simulink model "PVBOOSTCPL_MPPT"  (R2015a)
settings: Solver=ode3  StartTime=0.0  StopTime=inf  FixedStep=5e-5  RelTol=1e-3
libraries: powerlib x24, simulink x3, powerlib_meascontrol x2, fuzblock x1, simulink_extras x1, re_lib x1
settings Model: CovModelRefEnable=off  Creator=Nady  LastModifiedBy=ga63vey
settings DataIOCC: SaveFormat=Dataset
settings HardwareCC: ProdBitPerPointer=64  ProdLargestAtomicFloat=Float  ProdIntDivRoundTo=Zero  ProdEndianess=LittleEndian  ProdHWDeviceType=Specified
settings GRTTargetCC: GeneratePreprocessorConditionals=Use local settings

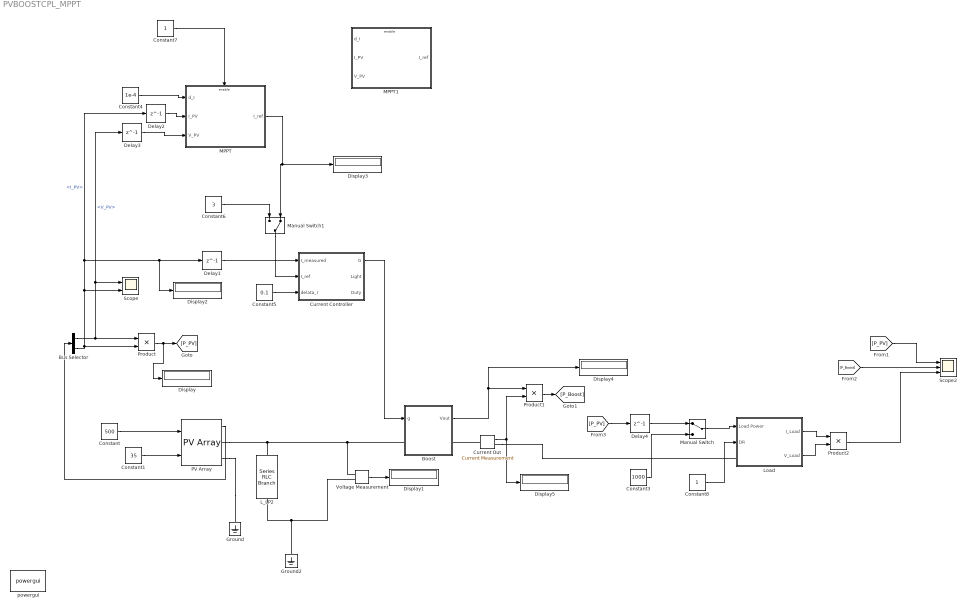
== system PVBOOSTCPL_MPPT ==
  Boost : Subsystem
  Bus Selector : BusSelector  OutputSignals=V_PV,I_PV
  Constant : Constant  Value=500
  Constant1 : Constant  Value=35
  Constant3 : Constant  Value=1000
  Constant4 : Constant  Value=1e-4
  Constant5 : Constant  Value=0.1
  Constant6 : Constant  Value=3
  Constant7 : Constant
  Constant8 : Constant
  Current Controller : Subsystem  TreatAsAtomicUnit=on
  Current Out : powerlib/Measurements/Current Measurement  PhasorSimulation=off  OutputType=Complex  PSBequivalent=0
  Delay{1..4} (4 alike) : Delay  DelayLength=1  InitialCondition=0
  Display{,1..5} (6 alike) : Display
  Ground : powerlib/Elements/Ground  LConnTagsString=a
  Ground2 : powerlib/Elements/Ground  LConnTagsString=a
  L_LP2 : powerlib/Elements/Series RLC Branch  LConnTagsString=__new0  RConnTagsString=__new0  BranchType=RC  Resistance=0.5  Inductance=0.0164  SetiL0=off  InitialCurrent=0  Capacitance=0.1  Setx0=off  InitialVoltage=0  Measurements=None
  Load : Subsystem
  MPPT : Subsystem
  MPPT1 : Subsystem
  Manual Switch : ManualSwitch
  Manual Switch1 : ManualSwitch  CurrentSetting=0
  PV Array : re_lib/Solar/PV Array  Npar=1  Nser=1  PlotType=array @ 1000 W/m2 & specified temperatures  S_vec="[ 1000  500  100 ]"  Temp_C_vec=[35]  ModuleName=Sun Earth Solar Power TDB125x125-36-P 80W  PlotWhenSelected=off  Pm=80.004  Ncell=36  Voc=21.9  Isc=5  Vm=17.7  Im=4.52  beta_Voc_pc=-0.32  alpha_Isc_pc=0.04  beta_Voc=-0.07008  alpha_Isc=0.002  IL=5.0238  I0=3.6974e-11  nI=0.92596  Rsh=70.2892  Rs=0.35567  BAL=off  Tc=1e-6  Tfilter=5e-5
  Product : Product
  Product1 : Product
  Product2 : Product
  Scope : Scope  NumInputPorts=2
      settings: YMin=-4.3176~-0.64549  YMax=38.86394~7.07339
  Scope2 : Scope  NumInputPorts=3
      settings: YMin=57~58~57  YMax=64~64~64  SaveName=ScopeData2
  Voltage Measurement : powerlib/Measurements/Voltage Measurement  PhasorSimulation=off  OutputType=Complex  PSBequivalent=0
  powergui : powerlib/powergui  Priority=1  SimulationMode=Discrete  SolverType=Tustin  SampleTime=50e-6  frequency=60  SPID=off  DisableSnubberDevices=off  DisableRonSwitches=off  DisableVfSwitches=off  SwTol=0  DisplayEquations=off  Interpol=off  methode=off  Ts=10  FunctionMessages=off  echomessages=off  HookPort=off  EnableUseOfTLC=off  x0status=blocks  frequencyindice=0  Pbase=100e6  ErrMax=1e-4  Iterations=50  UnitsV=kV  UnitsW=MW  buscounter=0  RestoreLinks=warning  ResistiveCurrentMeasurement=off  Frange=[0:2:500]  Ylog=off  Xlog=on  ShowGrid=off  save=off  variable=ZData  structure=0  ZoomFFT=off  StartTime=0.0  cycles=1  DisplayStyle=1  fundamental=60  FreqAxis=off  MaxFrequency=1000  frequencyindicesteady=1  RmsSteady=1  display=off
  wires:
  Constant/1 -> PV Array/1
  Constant1/1 -> PV Array/2
  PV Array/1 -> Bus Selector/1
  Bus Selector/1 -> Delay3/1, Scope/1, Product/1  "<V_PV>"
  Bus Selector/2 -> Delay2/1, Display2/1, Delay1/1, Scope/2, Product/2  "<I_PV>"
  Boost/1(Vout) -> Display4/1, Product1/1
  Current Out/1 -> Product1/2, Display5/1
  Product/1 -> Display/1, [P_PV]
  Product1/1 -> [P_Boost]
  Manual Switch/1 -> Load/1(Load Power)
  Constant3/1 -> Manual Switch/2
  [P_PV] -> Delay4/1
  Voltage Measurement/1 -> Display1/1
  Constant5/1 -> Current Controller/3(delata_I)
  Delay1/1 -> Current Controller/1(I_measured)
  Constant4/1 -> MPPT/1(d_I)
  Delay2/1 -> MPPT/2(I_PV)
  Delay3/1 -> MPPT/3(V_PV)
  Delay4/1 -> Manual Switch/1
  MPPT/1(I_ref) -> Display3/1, Manual Switch1/2
  Constant7/1 -> MPPT/Enable
  Constant6/1 -> Manual Switch1/1
  Manual Switch1/1 -> Current Controller/2(I_ref)
  Constant8/1 -> Load/2(DR)
  [P_PV] -> Scope2/1
  [P_Boost] -> Scope2/2
  Load/1(I_Load) -> Product2/1
  Load/2(V_Load) -> Product2/2
  Product2/1 -> Scope2/3
  Current Controller/1(G) -> Boost/1(g)
  connections:
  PV Array/RConn2 -- Ground/LConn1
  Current Out/LConn1 -- Boost/RConn1
  Ground2/LConn1 -- Voltage Measurement/LConn2 -- L_LP2/LConn1
  Current Out/RConn1 -- Load/LConn1
  PV Array/RConn1 -- Voltage Measurement/LConn1 -- Boost/LConn1 -- L_LP2/RConn1

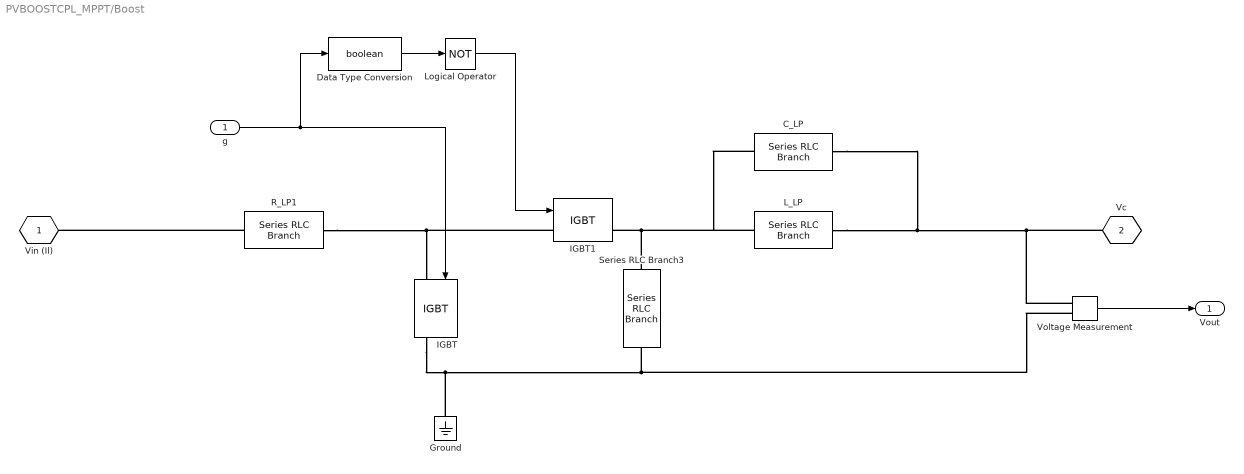
== system PVBOOSTCPL_MPPT/Boost ==
  g : Inport
  C_LP : powerlib/Elements/Series RLC Branch  LConnTagsString=__new0  RConnTagsString=__new0  BranchType=R  Resistance=10  Inductance=1e-3  SetiL0=off  InitialCurrent=0  Capacitance=0.004  Setx0=off  InitialVoltage=0  Measurements=None
  Data Type Conversion : DataTypeConversion  OutDataTypeStr=boolean
  Ground : powerlib/Elements/Ground  LConnTagsString=a
  IGBT : powerlib/Power Electronics/IGBT  Ron=0.001  Lon=0  Vf=1  Tf=1e-6  Tt=2e-6  IC=0  Rs=1e5  Cs=inf  Measurements=on
  IGBT1 : powerlib/Power Electronics/IGBT  Ron=0.001  Lon=0  Vf=1  Tf=1e-6  Tt=2e-6  IC=0  Rs=1e5  Cs=inf  Measurements=on
  L_LP : powerlib/Elements/Series RLC Branch  LConnTagsString=__new0  RConnTagsString=__new0  BranchType=L  Resistance=0.01  Inductance=0.0164  SetiL0=off  InitialCurrent=0  Capacitance=6e-2  Setx0=off  InitialVoltage=0  Measurements=None
  Logical Operator : Logic  Operator=NOT  AllPortsSameDT=off  OutDataTypeStr=boolean
  R_LP1 : powerlib/Elements/Series RLC Branch  LConnTagsString=__new0  RConnTagsString=__new0  BranchType=L  Resistance=0.01  Inductance=7e-3  SetiL0=off  InitialCurrent=0  Capacitance=6e-2  Setx0=off  InitialVoltage=0  Measurements=None
  Series RLC Branch3 : powerlib/Elements/Series RLC Branch  LConnTagsString=__new0  RConnTagsString=__new0  BranchType=RC  Resistance=0.1  Inductance=1e-3  SetiL0=off  InitialCurrent=0  Capacitance=6e-3  Setx0=off  InitialVoltage=0  Measurements=None
  Voltage Measurement : powerlib/Measurements/Voltage Measurement  PhasorSimulation=off  OutputType=Complex  PSBequivalent=0
  Vin (Il) : PMIOPort  Tag=PMCPort  Port=1  Side=Left
  Vc : PMIOPort  Tag=PMCPort  Port=2  Side=Right
  Vout : Outport
  wires:
  Voltage Measurement/1 -> Vout/1
  Data Type Conversion/1 -> Logical Operator/1
  Logical Operator/1 -> IGBT1/1
  g/1 -> Data Type Conversion/1, IGBT/1
  connections:
  IGBT/RConn1 -- Ground/LConn1 -- Voltage Measurement/LConn2 -- Series RLC Branch3/RConn1
  IGBT1/LConn1 -- R_LP1/LConn1 -- IGBT/LConn1
  R_LP1/RConn1 -- Vin (Il)/RConn1
  L_LP/LConn1 -- C_LP/LConn1 -- Voltage Measurement/LConn1 -- Vc/RConn1
  Series RLC Branch3/LConn1 -- C_LP/RConn1 -- L_LP/RConn1 -- IGBT1/RConn1

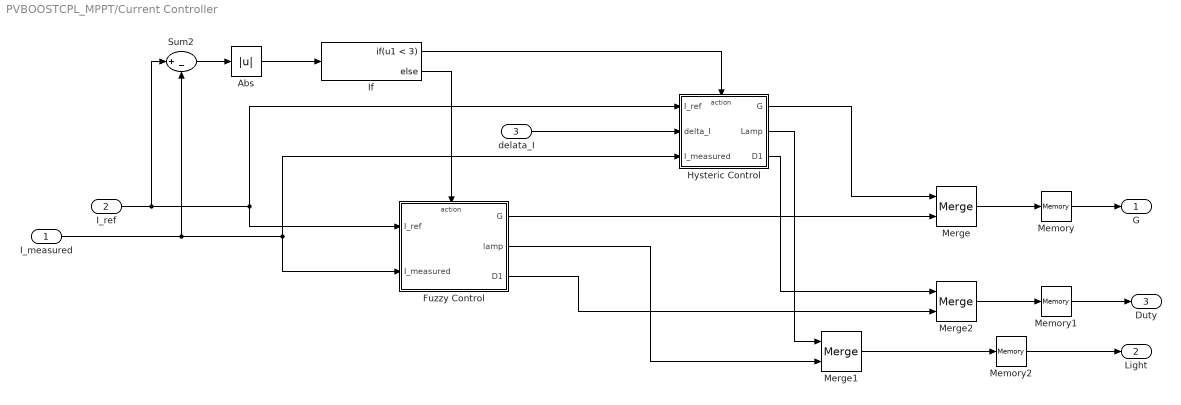
== system PVBOOSTCPL_MPPT/Current Controller ==
  I_measured : Inport  SampleTime=5e-5
  I_ref : Inport  Port=2  SampleTime=5e-5
  delata_I : Inport  Port=3
  Abs : Abs
  Fuzzy Control : Subsystem  TreatAsAtomicUnit=on
  Hysteric Control : Subsystem  TreatAsAtomicUnit=on
  If : If  IfExpression=u1 < 3
  Memory : Memory
  Memory1 : Memory
  Memory2 : Memory
  Merge : Merge
  Merge1 : Merge
  Merge2 : Merge
  Sum2 : Sum  Inputs=|+-
  G : Outport
  Light : Outport  Port=2
  Duty : Outport  Port=3
  wires:
  If/1 -> Hysteric Control/Action
  If/2 -> Fuzzy Control/Action
  I_ref/1 -> Sum2/1, Hysteric Control/1(I_ref), Fuzzy Control/1(I_ref)
  I_measured/1 -> Hysteric Control/3(I_measured), Fuzzy Control/2(I_measured), Sum2/2
  Fuzzy Control/1(G) -> Merge/2
  Merge/1 -> Memory/1
  delata_I/1 -> Hysteric Control/2(delta_I)
  Hysteric Control/1(G) -> Merge/1
  Hysteric Control/2(Lamp) -> Merge1/1
  Fuzzy Control/2(lamp) -> Merge1/2
  Merge1/1 -> Memory2/1
  Sum2/1 -> Abs/1
  Abs/1 -> If/1
  Fuzzy Control/3(D1) -> Merge2/2
  Merge2/1 -> Memory1/1
  Hysteric Control/3(D1) -> Merge2/1
  Memory/1 -> G/1
  Memory1/1 -> Duty/1
  Memory2/1 -> Light/1

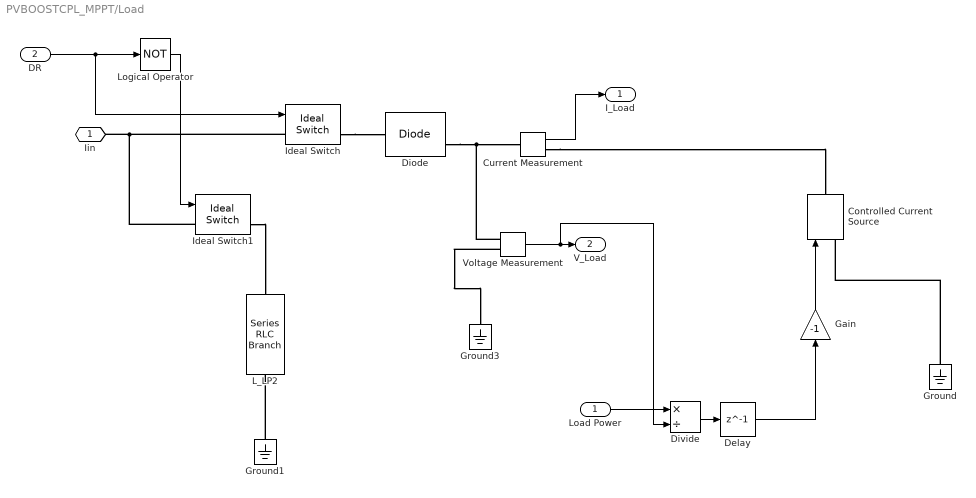
== system PVBOOSTCPL_MPPT/Load ==
  Load Power : Inport
  DR : Inport  Port=2
  Controlled Current Source : powerlib/Electrical Sources/Controlled Current Source  Initialize=on  Source_Type=AC  Amplitude=0  Phase=0  Frequency=0  Measurements=None
  Current Measurement : powerlib/Measurements/Current Measurement  PhasorSimulation=off  OutputType=Complex  PSBequivalent=0
  Delay : Delay  DelayLength=1
  Diode : powerlib/Power Electronics/Diode  Ron=0.001  Lon=0  Vf=0.8  IC=0  UseSnubber=off  Rs=500  Cs=250e-9  Measurements=on
  Divide : Product  Inputs=*/
  Gain : Gain  Gain=-1
  Ground : powerlib/Elements/Ground  LConnTagsString=a
  Ground1 : powerlib/Elements/Ground  LConnTagsString=a
  Ground3 : powerlib/Elements/Ground  LConnTagsString=a
  Ideal Switch : powerlib/Power Electronics/Ideal Switch  Ron=0.001  Lon=0  IC=0  Rs=1e5  Cs=inf  Measurements=on
  Ideal Switch1 : powerlib/Power Electronics/Ideal Switch  Ron=0.001  Lon=0  IC=0  Rs=1e5  Cs=inf  Measurements=on
  L_LP2 : powerlib/Elements/Series RLC Branch  LConnTagsString=__new0  RConnTagsString=__new0  BranchType=R  Resistance=1  Inductance=0.0164  SetiL0=off  InitialCurrent=0  Capacitance=0.1  Setx0=off  InitialVoltage=0  Measurements=None
  Logical Operator : Logic  Operator=NOT  AllPortsSameDT=off  OutDataTypeStr=boolean
  Voltage Measurement : powerlib/Measurements/Voltage Measurement  PhasorSimulation=off  OutputType=Complex  PSBequivalent=0
  Iin : PMIOPort  Port=1  Side=Left
  I_Load : Outport
  V_Load : Outport  Port=2
  wires:
  Current Measurement/1 -> I_Load/1
  Voltage Measurement/1 -> Divide/2, V_Load/1
  Load Power/1 -> Divide/1
  Gain/1 -> Controlled Current Source/1
  Divide/1 -> Delay/1
  Delay/1 -> Gain/1
  Logical Operator/1 -> Ideal Switch1/1
  DR/1 -> Ideal Switch/1, Logical Operator/1
  connections:
  Voltage Measurement/LConn1 -- Diode/RConn1 -- Current Measurement/LConn1
  Voltage Measurement/LConn2 -- Ground3/LConn1
  Ground/LConn1 -- Controlled Current Source/LConn1
  Current Measurement/RConn1 -- Controlled Current Source/RConn1
  Ideal Switch/LConn1 -- Ideal Switch1/LConn1 -- Iin/RConn1
  Ground1/LConn1 -- L_LP2/LConn1
  Ideal Switch/RConn1 -- Diode/LConn1
  Ideal Switch1/RConn1 -- L_LP2/RConn1

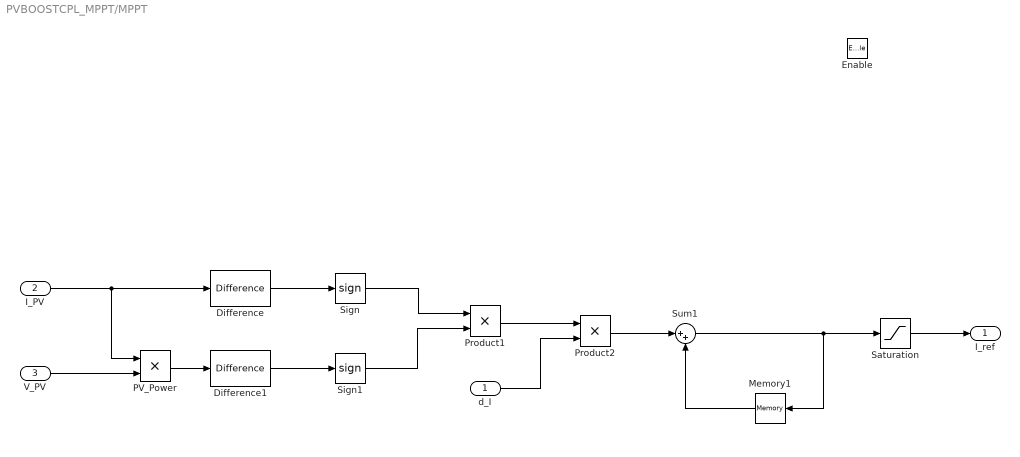
== system PVBOOSTCPL_MPPT/MPPT ==
  d_I : Inport
  I_PV : Inport  Port=2
  V_PV : Inport  Port=3
  Enable : EnablePort
  Difference : simulink/Discrete/Difference  ICPrevInput=0.0  InputProcessing=Inherited  OutMin=[]  OutMax=[]  OutDataType=fixdt(1, 16)  OutScaling=2^-10  DoSatur=off
  Difference1 : simulink/Discrete/Difference  ICPrevInput=0.0  InputProcessing=Inherited  OutMin=[]  OutMax=[]  OutDataType=fixdt(1, 16)  OutScaling=2^-10  DoSatur=off
  Memory1 : Memory
  PV_Power : Product
  Product1 : Product
  Product2 : Product
  Saturation : Saturate  UpperLimit=3.8  LowerLimit=0
  Sign : Signum
  Sign1 : Signum
  Sum1 : Sum  Inputs=|++
  I_ref : Outport
  wires:
  I_PV/1 -> PV_Power/1, Difference/1
  Difference/1 -> Sign/1
  V_PV/1 -> PV_Power/2
  PV_Power/1 -> Difference1/1
  Difference1/1 -> Sign1/1
  Sign/1 -> Product1/1
  Sign1/1 -> Product1/2
  Product1/1 -> Product2/1
  d_I/1 -> Product2/2
  Product2/1 -> Sum1/1
  Memory1/1 -> Sum1/2
  Sum1/1 -> Memory1/1, Saturation/1
  Saturation/1 -> I_ref/1

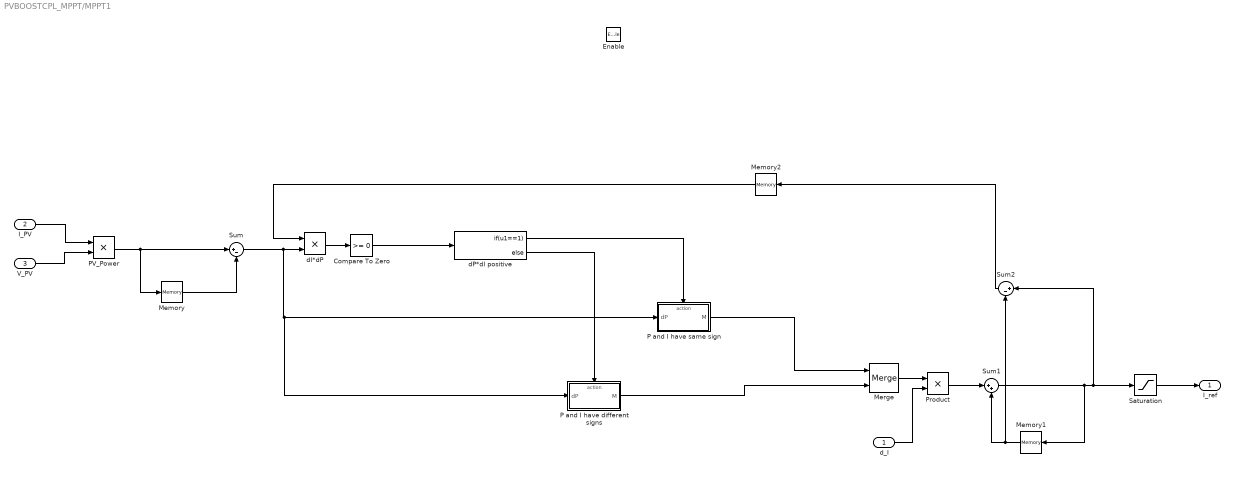
== system PVBOOSTCPL_MPPT/MPPT1 ==
  d_I : Inport
  I_PV : Inport  Port=2
  V_PV : Inport  Port=3
  Enable : EnablePort
  Compare To Zero : simulink/Logic and Bit Operations/Compare To Zero  relop=>=  OutDataTypeStr=boolean
  Memory : Memory
  Memory1 : Memory
  Memory2 : Memory
  Merge : Merge
  P and I have different signs : Subsystem  TreatAsAtomicUnit=on
  P and I have same sign : Subsystem  TreatAsAtomicUnit=on
  PV_Power : Product
  Product : Product
  Saturation : Saturate  UpperLimit=4.9  LowerLimit=0
  Sum : Sum  Inputs=|+-
  Sum1 : Sum  Inputs=|++
  Sum2 : Sum  Inputs=|+-
  dI*dP : Product
  dP*dI positive : If  IfExpression=u1==1
  I_ref : Outport
  wires:
  Saturation/1 -> I_ref/1
  Memory2/1 -> dI*dP/1
  Sum2/1 -> Memory2/1
  Memory1/1 -> Sum1/2, Sum2/2
  Product/1 -> Sum1/1
  Sum1/1 -> Saturation/1, Sum2/1, Memory1/1
  d_I/1 -> Product/2
  Merge/1 -> Product/1
  P and I have different signs/1(M) -> Merge/2
  P and I have same sign/1(M) -> Merge/1
  dP*dI positive/2 -> P and I have different signs/Action
  dP*dI positive/1 -> P and I have same sign/Action
  Compare To Zero/1 -> dP*dI positive/1
  dI*dP/1 -> Compare To Zero/1
  Sum/1 -> dI*dP/2, P and I have same sign/1(dP), P and I have different signs/1(dP)
  Memory/1 -> Sum/2
  PV_Power/1 -> Memory/1, Sum/1
  V_PV/1 -> PV_Power/2
  I_PV/1 -> PV_Power/1

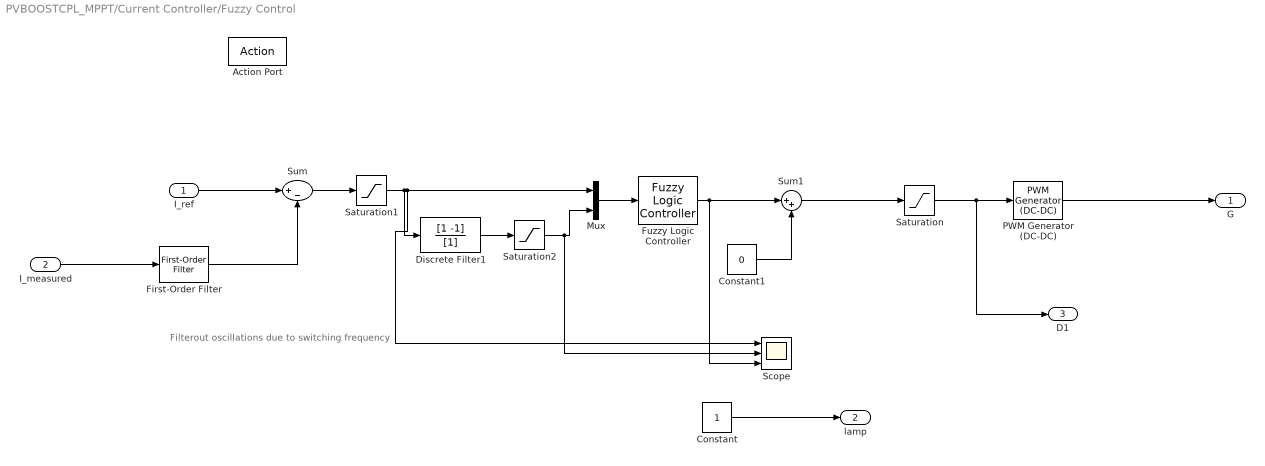
== system PVBOOSTCPL_MPPT/Current Controller/Fuzzy Control ==
  note: Filterout oscillations due to switching frequency
  I_ref : Inport
  I_measured : Inport  Port=2
  Action Port : ActionPort  ActionType=else
  Constant : Constant
  Constant1 : Constant  Value=0
  Discrete Filter1 : DiscreteFilter  Numerator=[1 -1]  Denominator=[1]
  First-Order Filter : powerlib_meascontrol/Filters/First-Order Filter  FilterType=Lowpass  Tc=1/8000  Ts=5e-5  Initialize=off  Vac_Init=[0, 0, 60]  Vdc_Init=0  PlotResponse=off  FreqRange="[0,  5000,  1]"
  Fuzzy Logic Controller : fuzblock/Fuzzy Logic  Controller  fis=ZIloop5
  Mux : Mux  Inputs=2
  PWM Generator (DC-DC) : powerlib_meascontrol/Pulse & Signal Generators/PWM Generator (DC-DC)  Fsw=10000  Ts=5e-5
  Saturation : Saturate  UpperLimit=0.8  LowerLimit=0
  Saturation1 : Saturate  UpperLimit=100  LowerLimit=-100
  Saturation2 : Saturate  UpperLimit=10  LowerLimit=-10
  Scope : Scope  NumInputPorts=3
      settings: YMin=-259.99999~-12.5~-0.04764  YMax=139.99989~12.5~0.84766
  Sum : Sum  Inputs=|+-
  Sum1 : Sum  Inputs=|++
  G : Outport
  lamp : Outport  Port=2  SourceOfInitialOutputValue=Input signal  InitialOutput=1
  D1 : Outport  Port=3
  wires:
  Mux/1 -> Fuzzy Logic Controller/1
  Fuzzy Logic Controller/1 -> Sum1/1, Scope/3
  I_ref/1 -> Sum/1
  Constant/1 -> lamp/1
  Saturation/1 -> D1/1, PWM Generator (DC-DC)/1
  PWM Generator (DC-DC)/1 -> G/1
  Sum/1 -> Saturation1/1
  Saturation1/1 -> Scope/1, Mux/1, Discrete Filter1/1
  Discrete Filter1/1 -> Saturation2/1
  Saturation2/1 -> Scope/2, Mux/2
  I_measured/1 -> First-Order Filter/1
  First-Order Filter/1 -> Sum/2
  Sum1/1 -> Saturation/1
  Constant1/1 -> Sum1/2

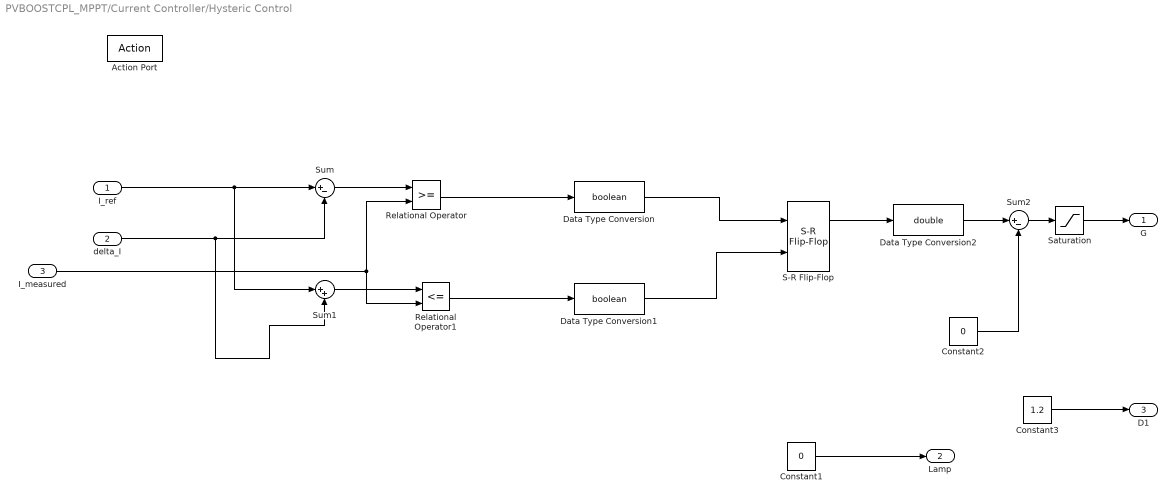
== system PVBOOSTCPL_MPPT/Current Controller/Hysteric Control ==
  I_ref : Inport
  delta_I : Inport  Port=2
  I_measured : Inport  Port=3
  Action Port : ActionPort  ActionType=then
  Constant1 : Constant  Value=0
  Constant2 : Constant  Value=0
  Constant3 : Constant  Value=1.2
  Data Type Conversion : DataTypeConversion  OutDataTypeStr=boolean
  Data Type Conversion1 : DataTypeConversion  OutDataTypeStr=boolean
  Data Type Conversion2 : DataTypeConversion  OutDataTypeStr=double
  Relational Operator : RelationalOperator  OutDataTypeStr=boolean  ZeroCross=off
  Relational Operator1 : RelationalOperator  Operator=<=  OutDataTypeStr=boolean  ZeroCross=off
  S-R Flip-Flop : simulink_extras/Flip Flops/S-R Flip-Flop  initial_condition=0
  Saturation : Saturate  UpperLimit=1  LowerLimit=0
  Sum : Sum  Inputs=|+-
  Sum1 : Sum  Inputs=|++
  Sum2 : Sum  Inputs=|+-
  G : Outport
  Lamp : Outport  Port=2  InitialOutput=1
  D1 : Outport  Port=3
  wires:
  I_ref/1 -> Sum1/1, Sum/1
  delta_I/1 -> Sum/2, Sum1/2
  Data Type Conversion/1 -> S-R Flip-Flop/1
  Data Type Conversion1/1 -> S-R Flip-Flop/2
  Sum/1 -> Relational Operator/1
  Relational Operator/1 -> Data Type Conversion/1
  Relational Operator1/1 -> Data Type Conversion1/1
  Sum1/1 -> Relational Operator1/1
  I_measured/1 -> Relational Operator/2, Relational Operator1/2
  Constant1/1 -> Lamp/1
  Data Type Conversion2/1 -> Sum2/1
  Constant2/1 -> Sum2/2
  Sum2/1 -> Saturation/1
  Saturation/1 -> G/1
  Constant3/1 -> D1/1
  S-R Flip-Flop/1 -> Data Type Conversion2/1

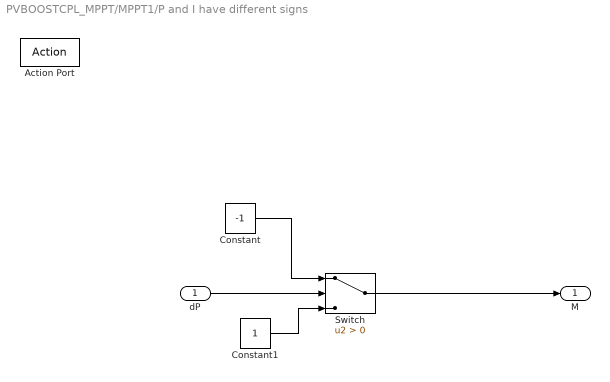
== system PVBOOSTCPL_MPPT/MPPT1/P and I have different signs ==
  dP : Inport
  Action Port : ActionPort  ActionType=else
  Constant : Constant  Value=-1
  Constant1 : Constant
  Switch : Switch  Criteria=u2 > Threshold
  M : Outport  InitialOutput=1
  wires:
  Switch/1 -> M/1
  Constant1/1 -> Switch/3
  Constant/1 -> Switch/1
  dP/1 -> Switch/2

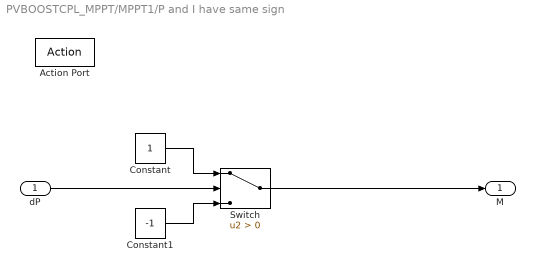
== system PVBOOSTCPL_MPPT/MPPT1/P and I have same sign ==
  dP : Inport
  Action Port : ActionPort  ActionType=then
  Constant : Constant
  Constant1 : Constant  Value=-1
  Switch : Switch  Criteria=u2 > Threshold
  M : Outport  InitialOutput=1
  wires:
  Switch/1 -> M/1
  Constant1/1 -> Switch/3
  Constant/1 -> Switch/1
  dP/1 -> Switch/2
